simulink model "Maze_haptic"  (Simulink 7.0)
settings: Solver=ode3  StartTime=0.0  StopTime=inf  FixedStep=0.01  RelTol=1e-3
values from neighbouring files (symbols this model uses):
  map_x = zeros(100,100)    [Make_Map.m]    (also in Make_Map_highrez.m = zeros(1000,1000))
  map_y = zeros(100,100)    [Make_Map.m]    (also in Make_Map_highrez.m = zeros(1000,1000))
libraries: quarc_library x1
settings Model: Creator=colinlea  LastModifiedBy=colinlea  SimulationMode=external  ExtModeTrigDuration=10000
settings SolverCC: PositivePriorityOrder=on
settings DataIOCC: ExternalInput=[map_x, map_y]
settings RTWCC: SystemTargetFile=quarc_windows.tlc  TemplateMakefile=quarc_default_tmf  Description=QuaRC Win32 Target  ProcessScript=quarc_windows_make_rtw_hook
settings STFCustomTargetCC: TargetPreCompLibLocation=C:\DOCUME~1\ALLUSE~1\APPLIC~1\QuaRC\lib\2007b\windows\release  GenFloatMathFcnCalls=ANSI_C  SystemTargetFile=quarc_windows.tlc
settings GRTTargetCC: TargetPreCompLibLocation=C:\DOCUME~1\ALLUSE~1\APPLIC~1\QuaRC\lib\2007b\windows\release  CompOptLevelCompliant=off  MatFileLogging=off  ExtMode=on  ExtModeMexFile=quarc_comm

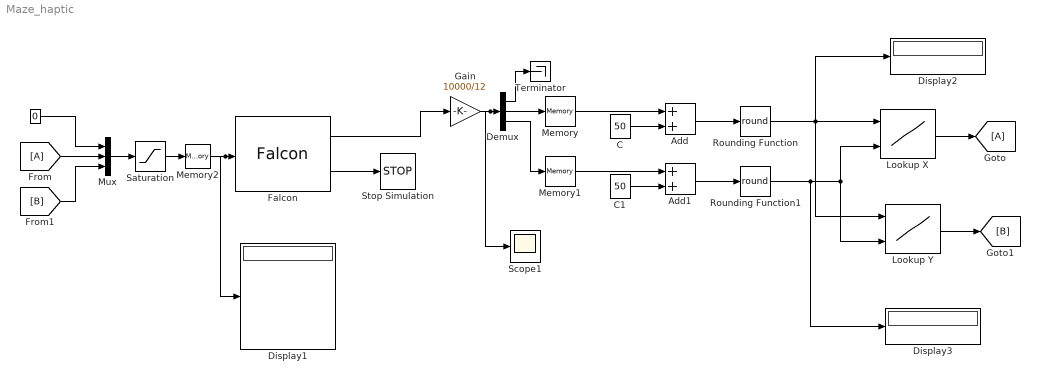
== system Maze_haptic ==
  "   " : Constant  Value=0  OutDataType=sfix(16)  OutScaling=2^0
  Add : Sum  OutDataType=sfix(16)  OutScaling=2^-10
  Add1 : Sum  OutDataType=sfix(16)  OutScaling=2^-10
  C : Constant  Value=50  OutDataType=sfix(16)  OutScaling=2^0
  C1 : Constant  Value=50  OutDataType=sfix(16)  OutScaling=2^0
  Demux : Demux  Outputs=3
  Display1 : Display
  Display2 : Display
  Display3 : Display
  Falcon : quarc_library/Devices/Third-Party/Novint/Falcon  sample_time=-1  show_calibrate=off
  Gain : Gain  Gain=10000/12  ParameterDataType=sfix(16)  ParameterScaling=2^0  OutDataType=sfix(16)  OutScaling=2^0
  Lookup X : Lookup2D  RowIndex=[1:1000]  ColumnIndex=[1:1000]  Table=map_y  LookUpMeth=Use Input Nearest  OutDataTypeMode=double  OutDataType=sfix(16)  OutScaling=2^0  RndMeth=Nearest  SaturateOnIntegerOverflow=on
  Lookup Y : Lookup2D  RowIndex=[1:1000]  ColumnIndex=[1:1000]  Table=map_x  LookUpMeth=Use Input Nearest  OutDataTypeMode=double  OutDataType=sfix(16)  OutScaling=2^0  RndMeth=Nearest  SaturateOnIntegerOverflow=on
  Memory : Memory  InheritSampleTime=on  LinearizeMemory=on  LinearizeAsDelay=on
  Memory1 : Memory  InheritSampleTime=on  LinearizeMemory=on  LinearizeAsDelay=on
  Memory2 : Memory  InheritSampleTime=on  LinearizeMemory=on  LinearizeAsDelay=on
  Mux : Mux  Inputs=3
  Rounding Function : Rounding  Operator=round
  Rounding Function1 : Rounding  Operator=round
  Saturation : Saturate  UpperLimit=5  LowerLimit=-5  OutDataType=sfix(16)  OutScaling=2^0
  Scope1 : Scope
      settings: YMin=-1.5e+022  YMax=1e+021
  Stop Simulation : Stop
  Terminator : Terminator
  wires:
  Gain/1 -> Demux/1, Scope1/1
  Falcon/1 -> Gain/1
  "   "/1 -> Mux/1
  [A] -> Mux/2
  [B] -> Mux/3
  Demux/2 -> Memory/1
  Demux/3 -> Memory1/1
  C/1 -> Add/2
  C1/1 -> Add1/2
  Add/1 -> Rounding Function/1
  Add1/1 -> Rounding Function1/1
  Falcon/2 -> Stop Simulation/1
  Lookup X/1 -> [A]
  Lookup Y/1 -> [B]
  Mux/1 -> Saturation/1
  Rounding Function/1 -> Lookup X/1, Lookup Y/1, Display2/1
  Rounding Function1/1 -> Lookup X/2, Lookup Y/2, Display3/1
  Saturation/1 -> Memory2/1
  Memory2/1 -> Display1/1, Falcon/1
  Memory/1 -> Add/1
  Memory1/1 -> Add1/1
  Demux/1 -> Terminator/1
